simulink subsystem "IR_LEDs"  (R2023a)
settings: Solver=VariableStepAuto  StartTime=0.0  StopTime=10.0  RelTol=1e-3
libraries: stm32f4xxblockslib x8
settings Model: Creator=JesseJabezArendse  LastModifiedBy=Dylan Howard

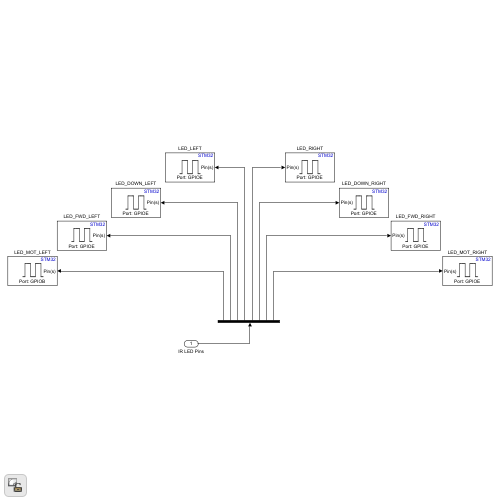
[thumbnail: Simulink's stored preview of the top-level diagram]
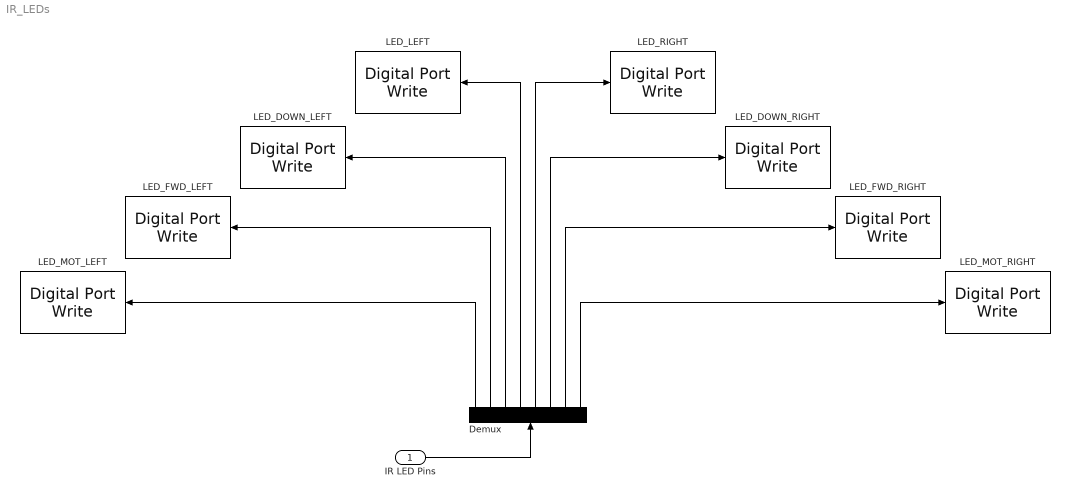
== system IR_LEDs ==
  IR LED Pins : Inport
  Demux : Demux  Outputs=8
  LED_DOWN_LEFT : stm32f4xxblockslib/Digital Port Write  PortName=GPIOE  PinNumber=9  ReadOperation=off  IOAsArray=on  EnableSimPort=off
      settings: LibrarySourceBlock=stm32l4xxblockslib/Digital Port Write
  LED_DOWN_RIGHT : stm32f4xxblockslib/Digital Port Write  PortName=GPIOE  PinNumber=14  ReadOperation=off  IOAsArray=on  EnableSimPort=off
      settings: LibrarySourceBlock=stm32l4xxblockslib/Digital Port Write
  LED_FWD_LEFT : stm32f4xxblockslib/Digital Port Write  PortName=GPIOE  PinNumber=8  ReadOperation=off  IOAsArray=on  EnableSimPort=off
      settings: LibrarySourceBlock=stm32l4xxblockslib/Digital Port Write
  LED_FWD_RIGHT : stm32f4xxblockslib/Digital Port Write  PortName=GPIOE  PinNumber=15  ReadOperation=off  IOAsArray=on  EnableSimPort=off
      settings: LibrarySourceBlock=stm32l4xxblockslib/Digital Port Write
  LED_LEFT : stm32f4xxblockslib/Digital Port Write  PortName=GPIOE  PinNumber=12  ReadOperation=off  IOAsArray=on  EnableSimPort=off
      settings: LibrarySourceBlock=stm32l4xxblockslib/Digital Port Write
  LED_MOT_LEFT : stm32f4xxblockslib/Digital Port Write  PortName=GPIOB  PinNumber=12  ReadOperation=off  IOAsArray=on  EnableSimPort=off
      settings: LibrarySourceBlock=stm32l4xxblockslib/Digital Port Write
  LED_MOT_RIGHT : stm32f4xxblockslib/Digital Port Write  PortName=GPIOE  PinNumber=13  ReadOperation=off  IOAsArray=on  EnableSimPort=off
      settings: LibrarySourceBlock=stm32l4xxblockslib/Digital Port Write
  LED_RIGHT : stm32f4xxblockslib/Digital Port Write  PortName=GPIOE  PinNumber=11  ReadOperation=off  IOAsArray=on  EnableSimPort=off
      settings: LibrarySourceBlock=stm32l4xxblockslib/Digital Port Write
  wires:
  Demux/1 -> LED_MOT_LEFT/1
  Demux/2 -> LED_FWD_LEFT/1
  Demux/4 -> LED_LEFT/1
  Demux/5 -> LED_RIGHT/1
  Demux/7 -> LED_FWD_RIGHT/1
  Demux/8 -> LED_MOT_RIGHT/1
  Demux/3 -> LED_DOWN_LEFT/1
  Demux/6 -> LED_DOWN_RIGHT/1
  IR LED Pins/1 -> Demux/1
